simulink model "AN_Simulink_Model_v1_fil"  (R2019b)
settings: Solver=VariableStepAuto  StartTime=0.0  StopTime=testtime  RelTol=1e-3
InitFcn:
  | AN_InitFcn_Callback
StopFcn:
  | AN_StopFcn_Callback
undefined symbols (not defined in the file or in its folder): tdres
libraries: hdlmdlgenlib x193, simulink x4, fillib x1, dspsrcs4 x1
(part 1 of 6)
settings Model: Creator=mblun  LastModifiedBy=t96f346
settings OptimizationCC: BlockReduction=off  ConditionallyExecuteInputs=off  DefaultParameterBehavior=Inlined
settings DebuggingCC: AlgebraicLoopMsg=error  InheritedTsInSrcMsg=none  UnderSpecifiedDimensionMsg=warning
settings HardwareCC: ProdBitPerPointer=32  ProdBitPerSizeT=32  ProdBitPerPtrDiffT=32  ProdLargestAtomicFloat=None  ProdIntDivRoundTo=Undefined  ProdEndianess=Unspecified  ProdWordSize=32  ProdHWDeviceType=ASIC/FPGA->ASIC/FPGA  TargetBitPerPointer=64  TargetBitPerSizeT=64  TargetBitPerPtrDiffT=64  TargetLongLongMode=on  TargetIntDivRoundTo=Zero  TargetEndianess=LittleEndian  TargetWordSize=64  TargetHWDeviceType=Custom Processor->MATLAB Host Computer  ProdEqTarget=off
settings SFSimCC: CustomCodeUndefinedFunction=UseInterfaceOnly

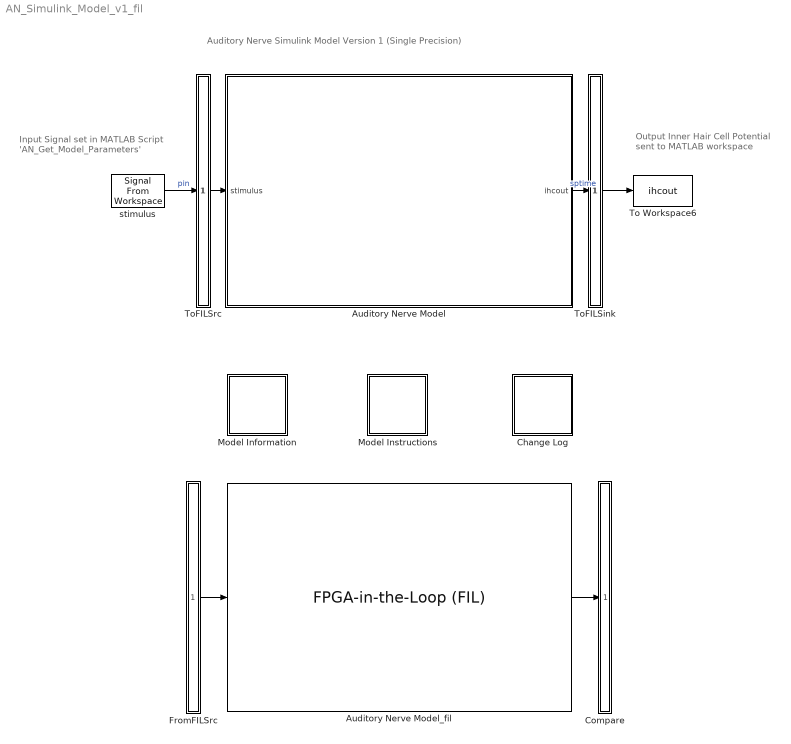
== system AN_Simulink_Model_v1_fil ==
  note: Input Signal set in MATLAB Script
      | 'AN_Get_Model_Parameters'
  note: Auditory Nerve Simulink Model Version 1 (Single Precision)
  note: Output Inner Hair Cell Potential
      | sent to MATLAB workspace
  Auditory Nerve Model : Subsystem
  Auditory Nerve Model_fil : fillib/FPGA-in-the-Loop (FIL)  ForceInterfaceUpdate=0.75839
      settings: SourceProductName=HDL Coder  SourceProductBaseCode=HD
  Change Log : Subsystem
  Compare : Subsystem
      mask Display: disp('')
  FromFILSrc : Subsystem
      mask Display: disp('')
  Model Information : Subsystem
  Model Instructions : Subsystem
  To Workspace6 : ToWorkspace  VariableName=ihcout  SampleTime=-1
      settings: Save2DSignal=2-D array (concatenate along first dimension)
  ToFILSink : Subsystem
      mask Display: disp('')
  ToFILSrc : Subsystem
      mask Display: disp('')
  "stimulus " : dspsrcs4/Signal From Workspace  X=RxSignal  Ts=tdres  nsamps=1  OutputAfterFinalValue=Setting to zero  ignoreOrWarnInputAndFrameLengths=off  OutputFrames=off
  wires:
  ToFILSrc/1(out1) -> Auditory Nerve Model/1(stimulus)
  Auditory Nerve Model/1(ihcout) -> ToFILSink/1(in1)  "sptime"
  "stimulus "/1 -> ToFILSrc/1(in1)  "pin"
  ToFILSink/1(out1) -> To Workspace6/1
  FromFILSrc/1(out1) -> Auditory Nerve Model_fil/1
  Auditory Nerve Model_fil/1 -> Compare/1(in1)

== system AN_Simulink_Model_v1_fil/Auditory Nerve Model ==
  stimulus : Inport  OutDataTypeStr=single  PortDimensions=1  SampleTime=2.08333333333333e-05
  C1 Chirp Filter : Subsystem
  C2 Wideband Filter : Subsystem
  CP Wideband Gammatone Filter : Subsystem
  Constant3 : Constant  Value=single(1.4316545724868774)  OutDataTypeStr=single  SampleTime=-1
  Constant4 : Constant  Value=single(0.0007758744177408516)  OutDataTypeStr=single  SampleTime=-1
  Middle Ear Filter : Subsystem
  Subsystem : Subsystem
  Subsystem1 : Subsystem
  ihcout : Outport  VectorParamsAs1DForOutWhenUnconnected=off
  wires:
  Subsystem1/1(tauc1) -> C1 Chirp Filter/2(tauc1)
  Subsystem/1(ihcout) -> ihcout/1
  Middle Ear Filter/1(output) -> C2 Wideband Filter/1(stimulus), C1 Chirp Filter/1(meout), CP Wideband Gammatone Filter/3(stimulus)
  Constant4/1 -> CP Wideband Gammatone Filter/2(tauwb)
  Constant3/1 -> CP Wideband Gammatone Filter/1(wbgain)
  CP Wideband Gammatone Filter/1(output1) -> Subsystem1/1(wbout)
  C2 Wideband Filter/1(output) -> Subsystem/1(C2filterout)
  C1 Chirp Filter/1(output) -> Subsystem/2(C1filterout)
  stimulus/1 -> Middle Ear Filter/1(stimulus)

== system AN_Simulink_Model_v1_fil/Change Log ==
  Change Log : simulink/Model-Wide Utilities/Model Info  Frame=on  DisplayStringWithTags=|  HorizontalTextAlignment=Left  LeftAlignmentValue=0.02
      | The following is the change log for the AN Simulink Model. Any major version changes should be 
      | documented and summarized below.
      | 
      | ------------------------------------------------------------------------------------------------------------------------------------
      | 
      | Version 1:
      | 	
      | 	- First Draft Version of Simulink Model by Matthew Blunt --- 08/07/2019
      | 
      | ------------------------------------------------------------------------------------------------------------------------------------
      | 
      | (Next Version Here)
      | 
      | 	- (Details and Changes Here)

== system AN_Simulink_Model_v1_fil/Compare ==
  in1 : Inport
  Assert_ihcout : Subsystem  mask{ToleranceValue=1e-07}
  CleanupScopes : Subsystem
      settings: OpenFcn=|
      | blkName = gcb; %self block
      | idx = regexp(blkName, '/CleanupScopes$', 'once');
      | blkParent = blkName(1:idx-1);
      | blks=find_system(blkParent, 'LookUnderMasks', 'all','blocktype', 'Scope');
      | for itr = 1:length(blks)
      | 	 hScopeCfg = get_param(blks{itr},'ScopeConfiguration');
      | 	 hScopeCfg.Visible = ~ hScopeCfg.Visible;
      | end
      | drawnow;
      mask Display: fprintf(message('hdlcoder:cosim:vnl_dblclick').getString());
  Enable : Subsystem
      settings: OpenFcn=|
      | blkName = gcb;
      | idx = regexp(blkName, '/Enable$', 'once');
      | blkParent = blkName(1:idx-1);
      | blks=find_system(blkParent, 'LookUnderMasks', 'all','blocktype', 'Assertion');
      | e = get_param(blks{1}, 'Enabled');
      | if strcmp(e, 'on'), f= 'off';, else, f = 'on';, end
      | for ii=1:length(blks), set_param(blks{ii}, 'Enabled', f);, end
      | set_param(gcb, 'MaskDisplay',['fprintf(message(''hdlcoder:cosim:vnl_dblclick_assertions'',','''',upper(e),'''',').getString())']);
      mask Display: fprintf(message('hdlcoder:cosim:vnl_dblclick_assertions','OFF').getString());
  wires:
  in1/1 -> Assert_ihcout/1(cosim)
  [out1] -> Assert_ihcout/2(dut)

== system AN_Simulink_Model_v1_fil/FromFILSrc ==
  dtc1 : DataTypeConversion  OutDataTypeStr=single  SaturateOnIntegerOverflow=on  RndMeth=Zero
  out1 : Outport
  wires:
  [in1] -> dtc1/1
  dtc1/1 -> out1/1

== system AN_Simulink_Model_v1_fil/Model Information ==
  "Model Information " : simulink/Model-Wide Utilities/Model Info  Frame=on  DisplayStringWithTags=|  HorizontalTextAlignment=Left  LeftAlignmentValue=0.02
      | Model Name: AN_Simulink_Model_v1
      | Created By: Matthew Blunt
      | Last Modification Date: 08/07/2019
      | Most Recently Modified By: Matthew Blunt
      | Model Version: 1
      | 
      | ------------------------------------------------------------------------------------------------------------------------------------
      | 
      | Description: This is a sample-based auditory nerve Simulink model, designed to closely replicate the 
      | auditory nerve model presented in the following publication:
      | 
      | 			Bruce, I.C., Erfani, Y., and Zilany, M.S.A. (2018). "A Phenomenological
      | 			model of the synapse between the inner hair cell and auditory nerve: 
      | 			Implications of limited neurotransmitter release sites," to appear in
      | 			Hearing Research. (Special Issue on "Computational Models in Hearing".)
      | 
      | It is important to also recognize the previous iterations of the phenomenological auditory 
      | nerve model, as they served as additional references during the design of the Simulink model.
      | 
      | ------------------------------------------------------------------------------------------------------------------------------------
      | 
      | This software was developed in conjunction with Flat Earth Inc
      | 
      | Copyright 2019 Flat Earth Inc
      | 
      | THE SOFTWARE IS PROVIDED "AS IS", WITHOUT WARRANTY OF ANY KIND, EXPRESS OR
      | IMPLIED, INCLUDING BUT NOT LIMITED TO THE WARRANTIES OF MERCHANTABILITY,
      | FITNESS FOR A PARTICULAR PURPOSE AND NONINFRINGEMENT. IN NO EVENT SHALL
      | THE AUTHORS OR COPYRIGHT HOLDERS BE LIABLE FOR ANY CLAIM, DAMAGES OR
      | OTHER LIABILITY, WHETHER IN AN ACTION OF CONTRACT, TORT OR OTHERWISE,
      | ARISING FROM, OUT OF OR IN CONNECTION WITH THE SOFTWARE OR THE USE OR
      | OTHER DEALINGS IN THE SOFTWARE.
      | 
      |    		Matthew Blunt
      |   		 Flat Earth Inc
      |    		985 Technology Blvd
      |    		Bozeman, MT 59718
      |    		support@flatearthinc.com

== system AN_Simulink_Model_v1_fil/Model Instructions ==
  "Model Instructions " : simulink/Model-Wide Utilities/Model Info  Frame=on  DisplayStringWithTags=|  HorizontalTextAlignment=Left  LeftAlignmentValue=0.02
      | The following is a full set of instructions outlining the necessary steps to be taken in order to run the 
      | AN Simulink Model. Instructions can also be found in the readme file found in the
      | AN_Simulink_Model_v1_Doubles folder.
      | 
      | ------------------------------------------------------------------------------------------------------------------------------------
      | 
      | ** Quick Start Instructions **
      | 
      | If the user desires to simply run the model as is, refer to the Quick Start
      | Instructions pdf, which gives a quick visual tutorial on running the Auditory
      | Nerve Simulink Model.
      | 
      | ------------------------------------------------------------------------------------------------------------------------------------
      | 
      | ** Modify Model Instructions **
      | 
      | If the user desires to make modifications to the model before runtime,
      | refer to the Modify Model Instructions pdf, which gives a quick visual
      | tutorial on modifying the Auditory Nerve Simulink Model.
      | 
      | ------------------------------------------------------------------------------------------------------------------------------------
      | 
      | ** Verify Model Instructions **
      | 
      | If the user desires to verify model functionality against the original 
      | model source code, instructions are listed below, as well as in the readme.txt file
      | 
      | 1. Make sure MATLAB R2019a and a compatible C compiler are downloaded on the
      | machine the model will be running on. The C compiler is needed for C functions
      | used in the test/verification process. The compiler used for testing was the
      | MinGW-w64 C/C++ Compiler. This can be easily accessed for free in the Add-On
      | Explorer found in the MATLAB home tab.
      | 
      | 2. Open the AN_Simulink_Model_v1_Doubles folder in MATLAB. This is necessary in
      | order for the Simulink model to interact with MATLAB.
      | 
      | 3. Edit model parameters, if necessary. This can be done by adjusting the
      | overall model parameters set in the AN_Set_Model_Parameters script, or adjusting
      | other parameters in the AN_Get_Model_Parameters script. Both scripts are found
      | in the AN_Simulink_Model_v1_Doubles folder.
      | 
      | 4. Set the 'verificationflag' boolean to 'true' in the AN_Set_Model_Parameters
      | script. This enables the model to run the comparison C/MATLAB source functions
      | which are compared to the Simulink Model.
      | 
      | 5. Run the model. This is done by simply clicking the green 'Run' button
      | located at the top panel of Simulink. In addition, the model can be stepped
      | through in increments, using the 'Step Through' button to the right of the
      | 'Run' button.

== system AN_Simulink_Model_v1_fil/ToFILSink ==
  in1 : Inport
  out1 : Outport
  tag scope: out1=global
  wires:
  in1/1 -> out1/1, [out1]

== system AN_Simulink_Model_v1_fil/ToFILSrc ==
  in1 : Inport
  out1 : Outport
  tag scope: in1=global
  wires:
  in1/1 -> out1/1, [in1]

== system AN_Simulink_Model_v1_fil/Auditory Nerve Model/C1 Chirp Filter ==
  meout : Inport  OutDataTypeStr=single  PortDimensions=1  SampleTime=2.08333333333333e-05
  tauc1 : Inport  Port=2  OutDataTypeStr=single  PortDimensions=1  SampleTime=2.08333333333333e-05
  C1 FIlter : Subsystem
  Calculate C1filterout : Subsystem
  Calculate rsigma : Subsystem
  Get C1 Coefficients : Subsystem
  To Workspace2 : ToWorkspace  VariableName=rsigma  SampleTime=-1
      settings: Save2DSignal=2-D array (concatenate along first dimension)
  output : Outport  VectorParamsAs1DForOutWhenUnconnected=off
  wires:
  Get C1 Coefficients/15(a1(5)) -> C1 FIlter/16(a1(5))
  Get C1 Coefficients/14(a1(3)) -> C1 FIlter/15(a1(3))
  Get C1 Coefficients/13(a1(1)) -> C1 FIlter/14(a1(1))
  Get C1 Coefficients/12(a2(1)) -> C1 FIlter/13(a2(1))
  Get C1 Coefficients/11(a2(3)) -> C1 FIlter/12(a2(3))
  Get C1 Coefficients/10(a2(5)) -> C1 FIlter/11(a2(5))
  Get C1 Coefficients/9(b2(1)) -> C1 FIlter/10(b2(1))
  Get C1 Coefficients/8(b2(3)) -> C1 FIlter/9(b2(3))
  Get C1 Coefficients/7(b2(5)) -> C1 FIlter/8(b2(5))
  Get C1 Coefficients/6(b1(1)) -> C1 FIlter/7(b1(1))
  Get C1 Coefficients/5(b1(3)) -> C1 FIlter/6(b1(3))
  Get C1 Coefficients/4(b1(5)) -> C1 FIlter/5(b1(5))
  Get C1 Coefficients/3(b0(1)) -> C1 FIlter/4(b0(1))
  Get C1 Coefficients/2(b0(3)) -> C1 FIlter/3(b0(3))
  Get C1 Coefficients/1(b0(5)) -> C1 FIlter/2(b0(5))
  Calculate rsigma/1(rsigma) -> Get C1 Coefficients/1(rsigma), To Workspace2/1
  Calculate C1filterout/1(C1filterout) -> output/1
  C1 FIlter/1(Out1) -> Calculate C1filterout/1(C1filterouttmp)
  tauc1/1 -> Calculate rsigma/1(tauc1)
  meout/1 -> C1 FIlter/1(meout)

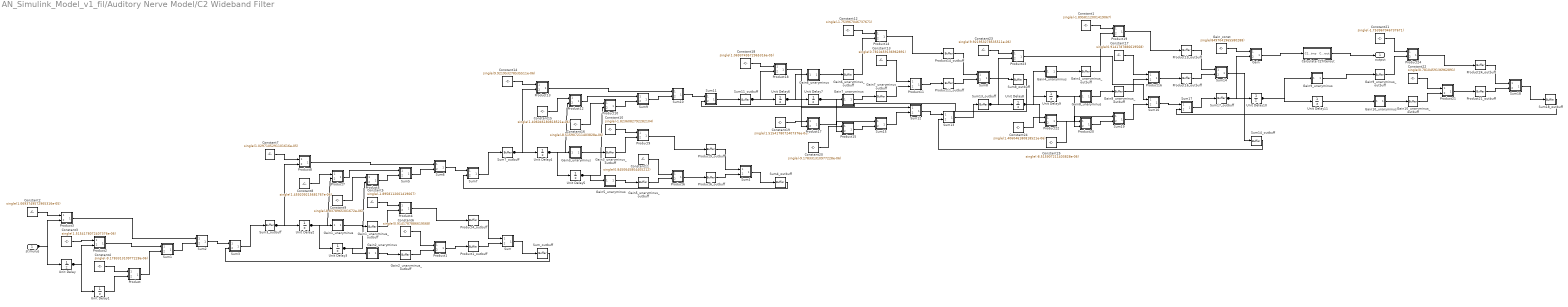
== system AN_Simulink_Model_v1_fil/Auditory Nerve Model/C2 Wideband Filter ==
  stimulus : Inport  OutDataTypeStr=single  PortDimensions=1  SampleTime=2.08333333333333e-05
  Calculate C2filterout : Subsystem
  Constant1 : Constant  Value=single(-1.8958112001419067)  OutDataTypeStr=single  SampleTime=-1
  Constant10 : Constant  Value=single(-1.8236082792282104)  OutDataTypeStr=single  SampleTime=-1
  Constant11 : Constant  Value=single(0.8450645804405212)  OutDataTypeStr=single  SampleTime=-1
  Constant12 : Constant  Value=single(-1.753967046737671)  OutDataTypeStr=single  SampleTime=-1
  Constant13 : Constant  Value=single(0.7810459136962891)  OutDataTypeStr=single  SampleTime=-1
  Constant14 : Constant  Value=single(9.921953278535511e-06)  OutDataTypeStr=single  SampleTime=-1
  Constant15 : Constant  Value=single(1.406046180818521e-06)  OutDataTypeStr=single  SampleTime=-1
  Constant16 : Constant  Value=single(-8.515907211403828e-06)  OutDataTypeStr=single  SampleTime=-1
  Constant17 : Constant  Value=single(0.9141787886619568)  OutDataTypeStr=single  SampleTime=-1
  Constant18 : Constant  Value=single(1.0693749572965316e-05)  OutDataTypeStr=single  SampleTime=-1
  Constant19 : Constant  Value=single(1.5154178072407376e-06)  OutDataTypeStr=single  SampleTime=-1
  Constant2 : Constant  Value=single(1.0693749572965316e-05)  OutDataTypeStr=single  SampleTime=-1
  Constant20 : Constant  Value=single(-9.178331310977228e-06)  OutDataTypeStr=single  SampleTime=-1
  Constant21 : Constant  Value=single(-1.753967046737671)  OutDataTypeStr=single  SampleTime=-1
  Constant22 : Constant  Value=single(0.7810459136962891)  OutDataTypeStr=single  SampleTime=-1
  Constant23 : Constant  Value=single(9.921953278535511e-06)  OutDataTypeStr=single  SampleTime=-1
  Constant24 : Constant  Value=single(1.406046180818521e-06)  OutDataTypeStr=single  SampleTime=-1
  Constant25 : Constant  Value=single(-8.515907211403828e-06)  OutDataTypeStr=single  SampleTime=-1
  Constant3 : Constant  Value=single(1.5154178072407376e-06)  OutDataTypeStr=single  SampleTime=-1
  Constant4 : Constant  Value=single(-9.178331310977228e-06)  OutDataTypeStr=single  SampleTime=-1
  Constant5 : Constant  Value=single(-1.8958112001419067)  OutDataTypeStr=single  SampleTime=-1
  Constant6 : Constant  Value=single(0.9141787886619568)  OutDataTypeStr=single  SampleTime=-1
  Constant7 : Constant  Value=single(1.0297105291101616e-05)  OutDataTypeStr=single  SampleTime=-1
  Constant8 : Constant  Value=single(1.459209215681767e-06)  OutDataTypeStr=single  SampleTime=-1
  Constant9 : Constant  Value=single(-8.8378965301672e-06)  OutDataTypeStr=single  SampleTime=-1
  Gain : Subsystem
      mask Display: disp('NFP\nmul');
  Gain10_unaryminus : Subsystem
      mask Display: disp('NFP\numinus');
  Gain10_unaryminus_outbuff : hdlmdlgenlib/Buffer
      settings: SourceProductName=Simulink  SourceProductBaseCode=SL
  Gain1_unaryminus : Subsystem
      mask Display: disp('NFP\numinus');
  Gain1_unaryminus_outbuff : hdlmdlgenlib/Buffer
      settings: SourceProductName=Simulink  SourceProductBaseCode=SL
  Gain2_unaryminus : Subsystem
      mask Display: disp('NFP\numinus');
  Gain2_unaryminus_outbuff : hdlmdlgenlib/Buffer
      settings: SourceProductName=Simulink  SourceProductBaseCode=SL
  Gain3_unaryminus : Subsystem
      mask Display: disp('NFP\numinus');
  Gain3_unaryminus_outbuff : hdlmdlgenlib/Buffer
      settings: SourceProductName=Simulink  SourceProductBaseCode=SL
  Gain4_unaryminus : Subsystem
      mask Display: disp('NFP\numinus');
  Gain4_unaryminus_outbuff : hdlmdlgenlib/Buffer
      settings: SourceProductName=Simulink  SourceProductBaseCode=SL
  Gain5_unaryminus : Subsystem
      mask Display: disp('NFP\numinus');
  Gain5_unaryminus_outbuff : hdlmdlgenlib/Buffer
      settings: SourceProductName=Simulink  SourceProductBaseCode=SL
  Gain6_unaryminus : Subsystem
      mask Display: disp('NFP\numinus');
  Gain6_unaryminus_outbuff : hdlmdlgenlib/Buffer
      settings: SourceProductName=Simulink  SourceProductBaseCode=SL
  Gain7_unaryminus : Subsystem
      mask Display: disp('NFP\numinus');
  Gain7_unaryminus_outbuff : hdlmdlgenlib/Buffer
      settings: SourceProductName=Simulink  SourceProductBaseCode=SL
  Gain8_unaryminus : Subsystem
      mask Display: disp('NFP\numinus');
  Gain8_unaryminus_outbuff : hdlmdlgenlib/Buffer
      settings: SourceProductName=Simulink  SourceProductBaseCode=SL
  Gain9_unaryminus : Subsystem
      mask Display: disp('NFP\numinus');
  Gain9_unaryminus_outbuff : hdlmdlgenlib/Buffer
      settings: SourceProductName=Simulink  SourceProductBaseCode=SL
  Gain_const : Constant  Value=single(8497041965580288)  OutDataTypeStr=single  SampleTime=-1
  Product : Subsystem
      mask Display: disp('NFP\nmul');
  Product1 : Subsystem
      mask Display: disp('NFP\nmul');
  Product10 : Subsystem
      mask Display: disp('NFP\nmul');
  Product11 : Subsystem
      mask Display: disp('NFP\nmul');
  Product11_outbuff : hdlmdlgenlib/Buffer
      settings: SourceProductName=Simulink  SourceProductBaseCode=SL
  Product12 : Subsystem
      mask Display: disp('NFP\nmul');
  Product13 : Subsystem
      mask Display: disp('NFP\nmul');
  Product14 : Subsystem
      mask Display: disp('NFP\nmul');
  Product14_outbuff : hdlmdlgenlib/Buffer
      settings: SourceProductName=Simulink  SourceProductBaseCode=SL
  Product15 : Subsystem
      mask Display: disp('NFP\nmul');
  Product16 : Subsystem
      mask Display: disp('NFP\nmul');
  Product16_outbuff : hdlmdlgenlib/Buffer
      settings: SourceProductName=Simulink  SourceProductBaseCode=SL
  Product17 : Subsystem
      mask Display: disp('NFP\nmul');
  Product18 : Subsystem
      mask Display: disp('NFP\nmul');
  Product19 : Subsystem
      mask Display: disp('NFP\nmul');
  Product19_outbuff : hdlmdlgenlib/Buffer
      settings: SourceProductName=Simulink  SourceProductBaseCode=SL
  Product1_outbuff : hdlmdlgenlib/Buffer
      settings: SourceProductName=Simulink  SourceProductBaseCode=SL
  Product2 : Subsystem
      mask Display: disp('NFP\nmul');
  Product20 : Subsystem
      mask Display: disp('NFP\nmul');
  Product21 : Subsystem
      mask Display: disp('NFP\nmul');
  Product21_outbuff : hdlmdlgenlib/Buffer
      settings: SourceProductName=Simulink  SourceProductBaseCode=SL
  Product22 : Subsystem
      mask Display: disp('NFP\nmul');
  Product23 : Subsystem
      mask Display: disp('NFP\nmul');
  Product24 : Subsystem
      mask Display: disp('NFP\nmul');
  Product24_outbuff : hdlmdlgenlib/Buffer
      settings: SourceProductName=Simulink  SourceProductBaseCode=SL
  Product3 : Subsystem
      mask Display: disp('NFP\nmul');
  Product4 : Subsystem
      mask Display: disp('NFP\nmul');
  Product4_outbuff : hdlmdlgenlib/Buffer
      settings: SourceProductName=Simulink  SourceProductBaseCode=SL
  Product5 : Subsystem
      mask Display: disp('NFP\nmul');
  Product6 : Subsystem
      mask Display: disp('NFP\nmul');
  Product6_outbuff : hdlmdlgenlib/Buffer
      settings: SourceProductName=Simulink  SourceProductBaseCode=SL
  Product7 : Subsystem
      mask Display: disp('NFP\nmul');
  Product8 : Subsystem
      mask Display: disp('NFP\nmul');
  Product9 : Subsystem
      mask Display: disp('NFP\nmul');
  Product9_outbuff : hdlmdlgenlib/Buffer
      settings: SourceProductName=Simulink  SourceProductBaseCode=SL
  Sum : Subsystem
      mask Display: disp('NFP\nadd');
  Sum1 : Subsystem
      mask Display: disp('NFP\nadd');
  Sum10 : Subsystem
      mask Display: disp('NFP\nadd');
  Sum11 : Subsystem
      mask Display: disp('NFP\nadd');
  Sum11_outbuff : hdlmdlgenlib/Buffer
      settings: SourceProductName=Simulink  SourceProductBaseCode=SL
  Sum12 : Subsystem
      mask Display: disp('NFP\nadd');
  Sum13 : Subsystem
      mask Display: disp('NFP\nadd');
  Sum13_outbuff : hdlmdlgenlib/Buffer
      settings: SourceProductName=Simulink  SourceProductBaseCode=SL
  Sum14 : Subsystem
      mask Display: disp('NFP\nadd');
  Sum14_outbuff : hdlmdlgenlib/Buffer
      settings: SourceProductName=Simulink  SourceProductBaseCode=SL
  Sum15 : Subsystem
      mask Display: disp('NFP\nadd');
  Sum16 : Subsystem
      mask Display: disp('NFP\nadd');
  Sum17 : Subsystem
      mask Display: disp('NFP\nadd');
  Sum17_outbuff : hdlmdlgenlib/Buffer
      settings: SourceProductName=Simulink  SourceProductBaseCode=SL
  Sum18 : Subsystem
      mask Display: disp('NFP\nadd');
  Sum18_outbuff : hdlmdlgenlib/Buffer
      settings: SourceProductName=Simulink  SourceProductBaseCode=SL
  Sum19 : Subsystem
      mask Display: disp('NFP\nadd');
  Sum2 : Subsystem
      mask Display: disp('NFP\nadd');
  Sum3 : Subsystem
      mask Display: disp('NFP\nadd');
  Sum3_outbuff : hdlmdlgenlib/Buffer
      settings: SourceProductName=Simulink  SourceProductBaseCode=SL
  Sum4 : Subsystem
      mask Display: disp('NFP\nadd');
  Sum4_outbuff : hdlmdlgenlib/Buffer
      settings: SourceProductName=Simulink  SourceProductBaseCode=SL
  Sum5 : Subsystem
      mask Display: disp('NFP\nadd');
  Sum6 : Subsystem
      mask Display: disp('NFP\nadd');
  Sum7 : Subsystem
      mask Display: disp('NFP\nadd');
  Sum7_outbuff : hdlmdlgenlib/Buffer
      settings: SourceProductName=Simulink  SourceProductBaseCode=SL
  Sum8 : Subsystem
      mask Display: disp('NFP\nadd');
  Sum8_outbuff : hdlmdlgenlib/Buffer
      settings: SourceProductName=Simulink  SourceProductBaseCode=SL
  Sum9 : Subsystem
      mask Display: disp('NFP\nadd');
  Sum_outbuff : hdlmdlgenlib/Buffer
      settings: SourceProductName=Simulink  SourceProductBaseCode=SL
  Unit Delay{,1..11} (12 alike) : UnitDelay  InitialCondition=single(0)  SampleTime=2.08333333333333e-05
  output : Outport  VectorParamsAs1DForOutWhenUnconnected=off
  wires:
  Gain/1(Out1) -> Calculate C2filterout/1(C2filterouttmp)
  Sum9/1(Out1) -> Sum10/2(In2)
  Sum8/1(Out1) -> Sum8_outbuff/1
  Sum7/1(Out1) -> Sum7_outbuff/1
  Sum6/1(Out1) -> Sum7/1(In1)
  Sum5/1(Out1) -> Sum6/2(In2)
  Sum4/1(Out1) -> Sum4_outbuff/1
  Sum3/1(Out1) -> Sum3_outbuff/1
  Sum2/1(Out1) -> Sum3/1(In1)
  Sum19/1(Out1) -> Sum16/2(In2)
  Sum18/1(Out1) -> Sum18_outbuff/1
  Sum17/1(Out1) -> Sum17_outbuff/1
  Sum16/1(Out1) -> Sum17/1(In1)
  Sum15/1(Out1) -> Sum12/2(In2)
  Sum14/1(Out1) -> Sum14_outbuff/1
  Sum13/1(Out1) -> Sum13_outbuff/1
  Sum12/1(Out1) -> Sum13/1(In1)
  Sum11/1(Out1) -> Sum11_outbuff/1
  Sum10/1(Out1) -> Sum11/1(In1)
  Sum1/1(Out1) -> Sum2/2(In2)
  Sum/1(Out1) -> Sum_outbuff/1
  Product9/1(Out1) -> Product9_outbuff/1
  Product8/1(Out1) -> Sum6/1(In1)
  Product7/1(Out1) -> Sum5/1(In1)
  Product6/1(Out1) -> Product6_outbuff/1
  Product5/1(Out1) -> Sum5/2(In2)
  Product4/1(Out1) -> Product4_outbuff/1
  Product3/1(Out1) -> Sum2/1(In1)
  Product24/1(Out1) -> Product24_outbuff/1
  Product23/1(Out1) -> Sum16/1(In1)
  Product22/1(Out1) -> Sum19/1(In1)
  Product21/1(Out1) -> Product21_outbuff/1
  Product20/1(Out1) -> Sum19/2(In2)
  Product2/1(Out1) -> Sum1/1(In1)
  Product19/1(Out1) -> Product19_outbuff/1
  Product18/1(Out1) -> Sum12/1(In1)
  Product17/1(Out1) -> Sum15/1(In1)
  Product16/1(Out1) -> Product16_outbuff/1
  Product15/1(Out1) -> Sum15/2(In2)
  Product14/1(Out1) -> Product14_outbuff/1
  Product13/1(Out1) -> Sum10/1(In1)
  Product12/1(Out1) -> Sum9/1(In1)
  Product11/1(Out1) -> Product11_outbuff/1
  Product10/1(Out1) -> Sum9/2(In2)
  Product1/1(Out1) -> Product1_outbuff/1
  Product/1(Out1) -> Sum1/2(In2)
  Gain9_unaryminus/1(Out1) -> Gain9_unaryminus_outbuff/1
  Gain8_unaryminus/1(Out1) -> Gain8_unaryminus_outbuff/1
  Gain7_unaryminus/1(Out1) -> Gain7_unaryminus_outbuff/1
  Gain6_unaryminus/1(Out1) -> Gain6_unaryminus_outbuff/1
  Gain5_unaryminus/1(Out1) -> Gain5_unaryminus_outbuff/1
  Gain4_unaryminus/1(Out1) -> Gain4_unaryminus_outbuff/1
  Gain3_unaryminus/1(Out1) -> Gain3_unaryminus_outbuff/1
  Gain2_unaryminus/1(Out1) -> Gain2_unaryminus_outbuff/1
  Gain10_unaryminus/1(Out1) -> Gain10_unaryminus_outbuff/1
  Gain1_unaryminus/1(Out1) -> Gain1_unaryminus_outbuff/1
  Gain_const/1 -> Gain/1(In1)
  Unit Delay9/1 -> Gain8_unaryminus/1(In1), Product20/2(In2)
  Unit Delay8/1 -> Unit Delay9/1, Gain4_unaryminus/1(In1), Product22/2(In2)
  Unit Delay7/1 -> Gain7_unaryminus/1(In1), Product15/2(In2)
  Unit Delay6/1 -> Unit Delay7/1, Gain6_unaryminus/1(In1), Product17/2(In2)
  Unit Delay5/1 -> Gain5_unaryminus/1(In1), Product10/2(In2)
  Unit Delay4/1 -> Unit Delay5/1, Gain3_unaryminus/1(In1), Product12/2(In2)
  Unit Delay3/1 -> Gain2_unaryminus/1(In1), Product5/2(In2)
  Unit Delay2/1 -> Unit Delay3/1, Gain1_unaryminus/1(In1), Product7/2(In2)
  Unit Delay11/1 -> Gain10_unaryminus/1(In1)
  Unit Delay10/1 -> Unit Delay11/1, Gain9_unaryminus/1(In1)
  Unit Delay1/1 -> Product/2(In2)
  Unit Delay/1 -> Unit Delay1/1, Product2/2(In2)
  Sum8_outbuff/1 -> Sum11/2(In2)
  Sum7_outbuff/1 -> Unit Delay4/1, Product13/2(In2)
  Sum4_outbuff/1 -> Sum7/2(In2)
  Sum3_outbuff/1 -> Unit Delay2/1, Product8/2(In2)
  Sum18_outbuff/1 -> Sum17/2(In2)
  Sum17_outbuff/1 -> Unit Delay10/1, Gain/2(In2)
  Sum14_outbuff/1 -> Sum13/2(In2)
  Sum13_outbuff/1 -> Unit Delay8/1, Product23/2(In2)
  Sum11_outbuff/1 -> Unit Delay6/1, Product18/2(In2)
  Sum_outbuff/1 -> Sum3/2(In2)
  Product9_outbuff/1 -> Sum4/1(In1)
  Product6_outbuff/1 -> Sum4/2(In2)
  Product4_outbuff/1 -> Sum/1(In1)
  Product24_outbuff/1 -> Sum18/1(In1)
  Product21_outbuff/1 -> Sum18/2(In2)
  Product19_outbuff/1 -> Sum14/1(In1)
  Product16_outbuff/1 -> Sum14/2(In2)
  Product14_outbuff/1 -> Sum8/1(In1)
  Product11_outbuff/1 -> Sum8/2(In2)
  Product1_outbuff/1 -> Sum/2(In2)
  Gain9_unaryminus_outbuff/1 -> Product24/2(In2)
  Gain8_unaryminus_outbuff/1 -> Product16/2(In2)
  Gain7_unaryminus_outbuff/1 -> Product11/2(In2)
  Gain6_unaryminus_outbuff/1 -> Product14/2(In2)
  Gain5_unaryminus_outbuff/1 -> Product6/2(In2)
  Gain4_unaryminus_outbuff/1 -> Product19/2(In2)
  Gain3_unaryminus_outbuff/1 -> Product9/2(In2)
  Gain2_unaryminus_outbuff/1 -> Product1/2(In2)
  Gain10_unaryminus_outbuff/1 -> Product21/2(In2)
  Gain1_unaryminus_outbuff/1 -> Product4/2(In2)
  Constant9/1 -> Product5/1(In1)
  Constant8/1 -> Product7/1(In1)
  Constant7/1 -> Product8/1(In1)
  Constant6/1 -> Product1/1(In1)
  Constant5/1 -> Product4/1(In1)
  Constant4/1 -> Product/1(In1)
  Constant3/1 -> Product2/1(In1)
  Constant25/1 -> Product20/1(In1)
  Constant24/1 -> Product22/1(In1)
  Constant23/1 -> Product23/1(In1)
  Constant22/1 -> Product21/1(In1)
  Constant21/1 -> Product24/1(In1)
  Constant20/1 -> Product15/1(In1)
  Constant2/1 -> Product3/1(In1)
  Constant19/1 -> Product17/1(In1)
  Constant18/1 -> Product18/1(In1)
  Constant17/1 -> Product16/1(In1)
  Constant16/1 -> Product10/1(In1)
  Constant15/1 -> Product12/1(In1)
  Constant14/1 -> Product13/1(In1)
  Constant13/1 -> Product11/1(In1)
  Constant12/1 -> Product14/1(In1)
  Constant11/1 -> Product6/1(In1)
  Constant10/1 -> Product9/1(In1)
  Constant1/1 -> Product19/1(In1)
  Calculate C2filterout/1(C2filterout) -> output/1
  stimulus/1 -> Unit Delay/1, Product3/2(In2)

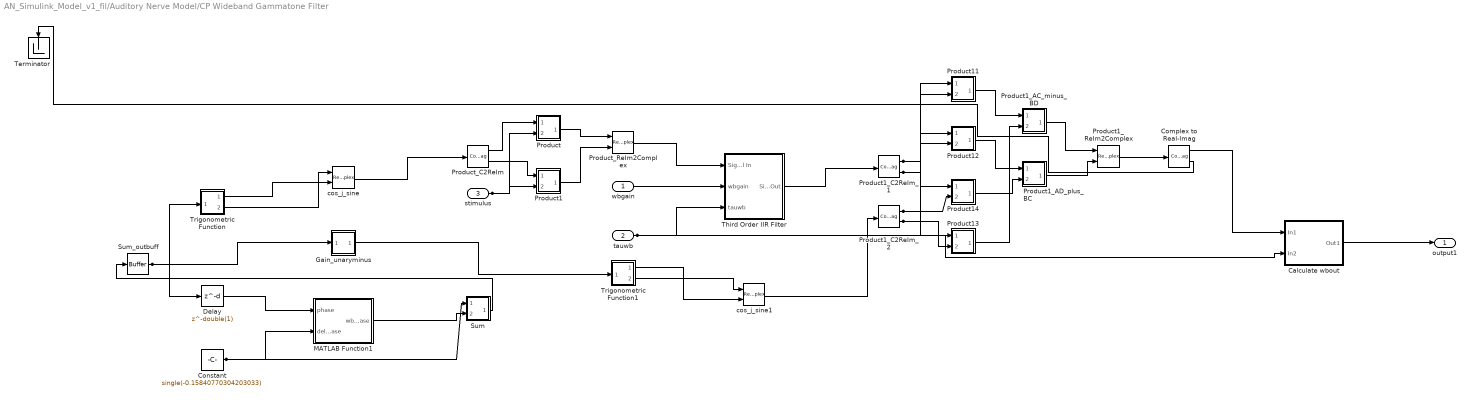
== system AN_Simulink_Model_v1_fil/Auditory Nerve Model/CP Wideband Gammatone Filter ==
  wbgain : Inport  OutDataTypeStr=single  PortDimensions=1  SampleTime=2.08333333333333e-05
  tauwb : Inport  Port=2  OutDataTypeStr=single  PortDimensions=1  SampleTime=2.08333333333333e-05
  stimulus : Inport  Port=3  OutDataTypeStr=single  PortDimensions=1  SampleTime=2.08333333333333e-05
  Calculate wbout : Subsystem
  Complex to Real-Imag : ComplexToRealImag  SampleTime=2.08333333333333e-05
  Constant : Constant  Value=single(-0.15840770304203033)  OutDataTypeStr=single  SampleTime=-1
  Delay : Delay  DelayLength=double(1)  InitialCondition=0  SampleTime=2.08333333333333e-05
  Gain_unaryminus : Subsystem
      mask Display: disp('NFP\numinus');
  MATLAB Function1 : Subsystem
  Product : Subsystem
      mask Display: disp('NFP\nmul');
  Product1 : Subsystem
      mask Display: disp('NFP\nmul');
  Product11 : Subsystem
      mask Display: disp('NFP\nmul');
  Product12 : Subsystem
      mask Display: disp('NFP\nmul');
  Product13 : Subsystem
      mask Display: disp('NFP\nmul');
  Product14 : Subsystem
      mask Display: disp('NFP\nmul');
  Product1_AC_minus_BD : Subsystem
      mask Display: disp('NFP\nadd');
  Product1_AD_plus_BC : Subsystem
      mask Display: disp('NFP\nadd');
  Product1_C2ReIm_1 : ComplexToRealImag  SampleTime=2.08333333333333e-05
  Product1_C2ReIm_2 : ComplexToRealImag  SampleTime=2.08333333333333e-05
  Product1_ReIm2Complex : RealImagToComplex  SampleTime=2.08333333333333e-05
  Product_C2ReIm : ComplexToRealImag  SampleTime=2.08333333333333e-05
  Product_ReIm2Complex : RealImagToComplex  SampleTime=2.08333333333333e-05
  Sum : Subsystem
      mask Display: disp('NFP\nadd');
  Sum_outbuff : hdlmdlgenlib/Buffer
      settings: SourceProductName=Simulink  SourceProductBaseCode=SL
  Terminator : Terminator
  Third Order IIR Filter : Subsystem
  Trigonometric Function : Subsystem
      mask Display: disp('NFP\ntrig2');
  Trigonometric Function1 : Subsystem
      mask Display: disp('NFP\ntrig2');
  cos_j_sine : RealImagToComplex  ConstantPart=single(0)  SampleTime=2.08333333333333e-05
  cos_j_sine1 : RealImagToComplex  ConstantPart=single(0)  SampleTime=2.08333333333333e-05
  output1 : Outport  VectorParamsAs1DForOutWhenUnconnected=off
  wires:
  Product1_AD_plus_BC/1(Out1) -> Product1_ReIm2Complex/2
  Product1_AC_minus_BD/1(Out1) -> Product1_ReIm2Complex/1
  Product14/1(Out1) -> Product1_AD_plus_BC/2(In2)
  Product13/1(Out1) -> Product1_AC_minus_BD/2(In2)
  Product12/1(Out1) -> Product1_AD_plus_BC/1(In1)
  Product11/1(Out1) -> Product1_AC_minus_BD/1(In1)
  Product1/1(Out1) -> Product_ReIm2Complex/2
  Product/1(Out1) -> Product_ReIm2Complex/1
  Trigonometric Function1/2(Out2) -> cos_j_sine1/1
  Trigonometric Function1/1(Out1) -> cos_j_sine1/2
  Trigonometric Function/2(Out2) -> cos_j_sine/1
  Trigonometric Function/1(Out1) -> cos_j_sine/2
  Sum/1(Out1) -> Sum_outbuff/1
  Gain_unaryminus/1(Out1) -> Trigonometric Function1/1(In1)
  Product1_C2ReIm_2/2 -> Product12/2(In2), Product13/2(In2)
  Product1_C2ReIm_2/1 -> Product11/2(In2), Product14/2(In2)
  Product1_C2ReIm_1/2 -> Product13/1(In1), Product14/1(In1)
  Product1_C2ReIm_1/1 -> Product11/1(In1), Product12/1(In1)
  Product_C2ReIm/2 -> Product1/1(In1)
  Product_C2ReIm/1 -> Product/1(In1)
  cos_j_sine1/1 -> Product1_C2ReIm_2/1
  cos_j_sine/1 -> Product_C2ReIm/1
  Third Order IIR Filter/1(Signal Out) -> Product1_C2ReIm_1/1
  Sum_outbuff/1 -> Delay/1, Gain_unaryminus/1(In1), Trigonometric Function/1(In1)
  Product1_ReIm2Complex/1 -> Complex to Real-Imag/1
  Product_ReIm2Complex/1 -> Third Order IIR Filter/1(Signal In)
  MATLAB Function1/1(wbphase) -> Sum/2(In2)
  Delay/1 -> MATLAB Function1/1(phase)
  Constant/1 -> MATLAB Function1/2(delta_phase), Sum/1(In1)
  Complex to Real-Imag/2 -> Terminator/1
  Complex to Real-Imag/1 -> Calculate wbout/1(In1)
  Calculate wbout/1(Out1) -> output1/1
  stimulus/1 -> Product/2(In2), Product1/2(In2)
  tauwb/1 -> Third Order IIR Filter/3(tauwb), Calculate wbout/2(In2)
  wbgain/1 -> Third Order IIR Filter/2(wbgain)

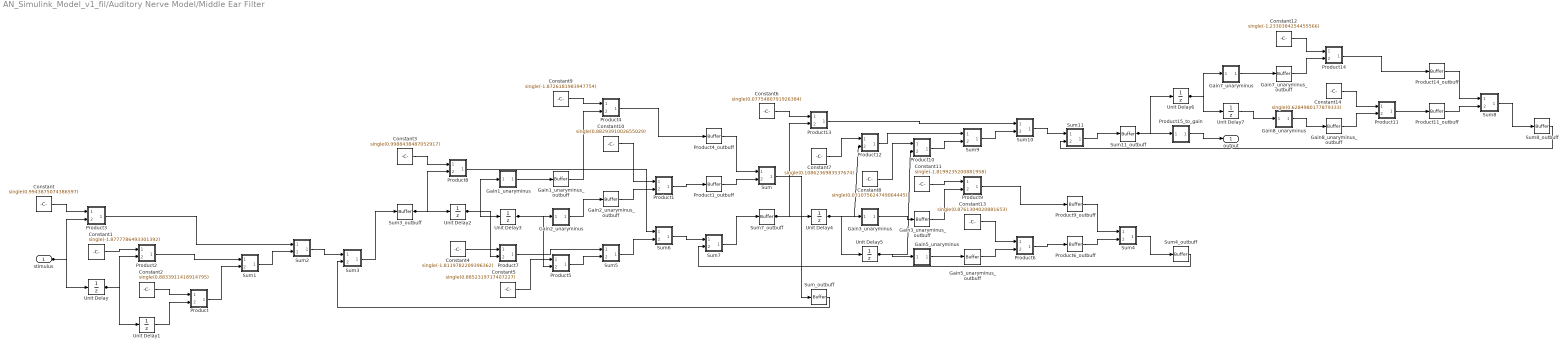
== system AN_Simulink_Model_v1_fil/Auditory Nerve Model/Middle Ear Filter ==
  stimulus : Inport  OutDataTypeStr=single  PortDimensions=1  SampleTime=2.08333333333333e-05
  Constant : Constant  Value=single(0.9943875074386597)  OutDataTypeStr=single  SampleTime=-1
  Constant1 : Constant  Value=single(-1.8777786493301392)  OutDataTypeStr=single  SampleTime=-1
  Constant10 : Constant  Value=single(0.8829391002655029)  OutDataTypeStr=single  SampleTime=-1
  Constant11 : Constant  Value=single(-1.8199235200881958)  OutDataTypeStr=single  SampleTime=-1
  Constant12 : Constant  Value=single(-1.2330384254455566)  OutDataTypeStr=single  SampleTime=-1
  Constant13 : Constant  Value=single(0.8761304020881653)  OutDataTypeStr=single  SampleTime=-1
  Constant14 : Constant  Value=single(0.6284980177879333)  OutDataTypeStr=single  SampleTime=-1
  Constant2 : Constant  Value=single(0.8833911418914795)  OutDataTypeStr=single  SampleTime=-1
  Constant3 : Constant  Value=single(0.9988438487052917)  OutDataTypeStr=single  SampleTime=-1
  Constant4 : Constant  Value=single(-1.8119782209396362)  OutDataTypeStr=single  SampleTime=-1
  Constant5 : Constant  Value=single(0.8852319717407227)  OutDataTypeStr=single  SampleTime=-1
  Constant6 : Constant  Value=single(0.0775480791926384)  OutDataTypeStr=single  SampleTime=-1
  Constant7 : Constant  Value=single(0.1086236983537674)  OutDataTypeStr=single  SampleTime=-1
  Constant8 : Constant  Value=single(0.031075624749064445)  OutDataTypeStr=single  SampleTime=-1
  Constant9 : Constant  Value=single(-1.8726181983947754)  OutDataTypeStr=single  SampleTime=-1
  Gain1_unaryminus : Subsystem
      mask Display: disp('NFP\numinus');
  Gain1_unaryminus_outbuff : hdlmdlgenlib/Buffer
      settings: SourceProductName=Simulink  SourceProductBaseCode=SL
  Gain2_unaryminus : Subsystem
      mask Display: disp('NFP\numinus');
  Gain2_unaryminus_outbuff : hdlmdlgenlib/Buffer
      settings: SourceProductName=Simulink  SourceProductBaseCode=SL
  Gain3_unaryminus : Subsystem
      mask Display: disp('NFP\numinus');
  Gain3_unaryminus_outbuff : hdlmdlgenlib/Buffer
      settings: SourceProductName=Simulink  SourceProductBaseCode=SL
  Gain5_unaryminus : Subsystem
      mask Display: disp('NFP\numinus');
  Gain5_unaryminus_outbuff : hdlmdlgenlib/Buffer
      settings: SourceProductName=Simulink  SourceProductBaseCode=SL
  Gain7_unaryminus : Subsystem
      mask Display: disp('NFP\numinus');
  Gain7_unaryminus_outbuff : hdlmdlgenlib/Buffer
      settings: SourceProductName=Simulink  SourceProductBaseCode=SL
  Gain8_unaryminus : Subsystem
      mask Display: disp('NFP\numinus');
  Gain8_unaryminus_outbuff : hdlmdlgenlib/Buffer
      settings: SourceProductName=Simulink  SourceProductBaseCode=SL
  Product : Subsystem
      mask Display: disp('NFP\nmul');
  Product1 : Subsystem
      mask Display: disp('NFP\nmul');
  Product10 : Subsystem
      mask Display: disp('NFP\nmul');
  Product11 : Subsystem
      mask Display: disp('NFP\nmul');
  Product11_outbuff : hdlmdlgenlib/Buffer
      settings: SourceProductName=Simulink  SourceProductBaseCode=SL
  Product12 : Subsystem
      mask Display: disp('NFP\nmul');
  Product13 : Subsystem
      mask Display: disp('NFP\nmul');
  Product14 : Subsystem
      mask Display: disp('NFP\nmul');
  Product14_outbuff : hdlmdlgenlib/Buffer
      settings: SourceProductName=Simulink  SourceProductBaseCode=SL
  Product15_to_gain : Subsystem
      mask Display: disp('NFP\ngain_pow2');
  Product1_outbuff : hdlmdlgenlib/Buffer
      settings: SourceProductName=Simulink  SourceProductBaseCode=SL
  Product2 : Subsystem
      mask Display: disp('NFP\nmul');
  Product3 : Subsystem
      mask Display: disp('NFP\nmul');
  Product4 : Subsystem
      mask Display: disp('NFP\nmul');
  Product4_outbuff : hdlmdlgenlib/Buffer
      settings: SourceProductName=Simulink  SourceProductBaseCode=SL
  Product5 : Subsystem
      mask Display: disp('NFP\nmul');
  Product6 : Subsystem
      mask Display: disp('NFP\nmul');
  Product6_outbuff : hdlmdlgenlib/Buffer
      settings: SourceProductName=Simulink  SourceProductBaseCode=SL
  Product7 : Subsystem
      mask Display: disp('NFP\nmul');
  Product8 : Subsystem
      mask Display: disp('NFP\nmul');
  Product9 : Subsystem
      mask Display: disp('NFP\nmul');
  Product9_outbuff : hdlmdlgenlib/Buffer
      settings: SourceProductName=Simulink  SourceProductBaseCode=SL
  Sum : Subsystem
      mask Display: disp('NFP\nadd');
  Sum1 : Subsystem
      mask Display: disp('NFP\nadd');
  Sum10 : Subsystem
      mask Display: disp('NFP\nadd');
  Sum11 : Subsystem
      mask Display: disp('NFP\nadd');
  Sum11_outbuff : hdlmdlgenlib/Buffer
      settings: SourceProductName=Simulink  SourceProductBaseCode=SL
  Sum2 : Subsystem
      mask Display: disp('NFP\nadd');
  Sum3 : Subsystem
      mask Display: disp('NFP\nadd');
  Sum3_outbuff : hdlmdlgenlib/Buffer
      settings: SourceProductName=Simulink  SourceProductBaseCode=SL
  Sum4 : Subsystem
      mask Display: disp('NFP\nadd');
  Sum4_outbuff : hdlmdlgenlib/Buffer
      settings: SourceProductName=Simulink  SourceProductBaseCode=SL
  Sum5 : Subsystem
      mask Display: disp('NFP\nadd');
  Sum6 : Subsystem
      mask Display: disp('NFP\nadd');
  Sum7 : Subsystem
      mask Display: disp('NFP\nadd');
  Sum7_outbuff : hdlmdlgenlib/Buffer
      settings: SourceProductName=Simulink  SourceProductBaseCode=SL
  Sum8 : Subsystem
      mask Display: disp('NFP\nadd');
  Sum8_outbuff : hdlmdlgenlib/Buffer
      settings: SourceProductName=Simulink  SourceProductBaseCode=SL
  Sum9 : Subsystem
      mask Display: disp('NFP\nadd');
  Sum_outbuff : hdlmdlgenlib/Buffer
      settings: SourceProductName=Simulink  SourceProductBaseCode=SL
  Unit Delay{,1..7} (8 alike) : UnitDelay  InitialCondition=single(0)  SampleTime=2.08333333333333e-05
  output : Outport  VectorParamsAs1DForOutWhenUnconnected=off
  wires:
  Product15_to_gain/1(Out1) -> output/1
  Sum9/1(Out1) -> Sum10/2(In2)
  Sum8/1(Out1) -> Sum8_outbuff/1
  Sum7/1(Out1) -> Sum7_outbuff/1
  Sum6/1(Out1) -> Sum7/1(In1)
  Sum5/1(Out1) -> Sum6/2(In2)
  Sum4/1(Out1) -> Sum4_outbuff/1
  Sum3/1(Out1) -> Sum3_outbuff/1
  Sum2/1(Out1) -> Sum3/1(In1)
  Sum11/1(Out1) -> Sum11_outbuff/1
  Sum10/1(Out1) -> Sum11/1(In1)
  Sum1/1(Out1) -> Sum2/2(In2)
  Sum/1(Out1) -> Sum_outbuff/1
  Product9/1(Out1) -> Product9_outbuff/1
  Product8/1(Out1) -> Sum6/1(In1)
  Product7/1(Out1) -> Sum5/1(In1)
  Product6/1(Out1) -> Product6_outbuff/1
  Product5/1(Out1) -> Sum5/2(In2)
  Product4/1(Out1) -> Product4_outbuff/1
  Product3/1(Out1) -> Sum2/1(In1)
  Product2/1(Out1) -> Sum1/1(In1)
  Product14/1(Out1) -> Product14_outbuff/1
  Product13/1(Out1) -> Sum10/1(In1)
  Product12/1(Out1) -> Sum9/1(In1)
  Product11/1(Out1) -> Product11_outbuff/1
  Product10/1(Out1) -> Sum9/2(In2)
  Product1/1(Out1) -> Product1_outbuff/1
  Product/1(Out1) -> Sum1/2(In2)
  Gain8_unaryminus/1(Out1) -> Gain8_unaryminus_outbuff/1
  Gain7_unaryminus/1(Out1) -> Gain7_unaryminus_outbuff/1
  Gain5_unaryminus/1(Out1) -> Gain5_unaryminus_outbuff/1
  Gain3_unaryminus/1(Out1) -> Gain3_unaryminus_outbuff/1
  Gain2_unaryminus/1(Out1) -> Gain2_unaryminus_outbuff/1
  Gain1_unaryminus/1(Out1) -> Gain1_unaryminus_outbuff/1
  Unit Delay7/1 -> Gain8_unaryminus/1(In1)
  Unit Delay6/1 -> Unit Delay7/1, Gain7_unaryminus/1(In1)
  Unit Delay5/1 -> Gain5_unaryminus/1(In1), Product10/2(In2)
  Unit Delay4/1 -> Unit Delay5/1, Gain3_unaryminus/1(In1), Product12/2(In2)
  Unit Delay3/1 -> Gain2_unaryminus/1(In1), Product5/2(In2)
  Unit Delay2/1 -> Unit Delay3/1, Gain1_unaryminus/1(In1), Product7/2(In2)
  Unit Delay1/1 -> Product/2(In2)
  Unit Delay/1 -> Unit Delay1/1, Product2/2(In2)
  Sum8_outbuff/1 -> Sum11/2(In2)
  Sum7_outbuff/1 -> Unit Delay4/1, Product13/2(In2)
  Sum4_outbuff/1 -> Sum7/2(In2)
  Sum3_outbuff/1 -> Unit Delay2/1, Product8/2(In2)
  Sum11_outbuff/1 -> Unit Delay6/1, Product15_to_gain/1(In1)
  Sum_outbuff/1 -> Sum3/2(In2)
  Product9_outbuff/1 -> Sum4/1(In1)
  Product6_outbuff/1 -> Sum4/2(In2)
  Product4_outbuff/1 -> Sum/1(In1)
  Product14_outbuff/1 -> Sum8/1(In1)
  Product11_outbuff/1 -> Sum8/2(In2)
  Product1_outbuff/1 -> Sum/2(In2)
  Gain8_unaryminus_outbuff/1 -> Product11/2(In2)
  Gain7_unaryminus_outbuff/1 -> Product14/2(In2)
  Gain5_unaryminus_outbuff/1 -> Product6/2(In2)
  Gain3_unaryminus_outbuff/1 -> Product9/2(In2)
  Gain2_unaryminus_outbuff/1 -> Product1/2(In2)
  Gain1_unaryminus_outbuff/1 -> Product4/2(In2)
  Constant9/1 -> Product4/1(In1)
  Constant8/1 -> Product10/1(In1)
  Constant7/1 -> Product12/1(In1)
  Constant6/1 -> Product13/1(In1)
  Constant5/1 -> Product5/1(In1)
  Constant4/1 -> Product7/1(In1)
  Constant3/1 -> Product8/1(In1)
  Constant2/1 -> Product/1(In1)
  Constant14/1 -> Product11/1(In1)
  Constant13/1 -> Product6/1(In1)
  Constant12/1 -> Product14/1(In1)
  Constant11/1 -> Product9/1(In1)
  Constant10/1 -> Product1/1(In1)
  Constant1/1 -> Product2/1(In1)
  Constant/1 -> Product3/1(In1)
  stimulus/1 -> Unit Delay/1, Product3/2(In2)

== system AN_Simulink_Model_v1_fil/Auditory Nerve Model/Subsystem ==
  C2filterout : Inport  OutDataTypeStr=single  PortDimensions=1  SampleTime=2.08333333333333e-05
  C1filterout : Inport  Port=2  OutDataTypeStr=single  PortDimensions=1  SampleTime=2.08333333333333e-05
  IHC C1 NL Logarithmic Function : Subsystem
  IHC C2 NL Logarithmic Function : Subsystem
  IHC LP Filter : Subsystem
  Sum1 : Subsystem
      mask Display: disp('NFP\nadd');
  ihcout : Outport  VectorParamsAs1DForOutWhenUnconnected=off
  wires:
  Sum1/1(Out1) -> IHC LP Filter/1(stimulus)
  IHC LP Filter/1(output) -> ihcout/1
  IHC C2 NL Logarithmic Function/1(output) -> Sum1/1(In1)
  IHC C1 NL Logarithmic Function/1(output) -> Sum1/2(In2)
  C1filterout/1 -> IHC C1 NL Logarithmic Function/1(stimulus)
  C2filterout/1 -> IHC C2 NL Logarithmic Function/1(stimulus)

== system AN_Simulink_Model_v1_fil/Auditory Nerve Model/Subsystem1 ==
  wbout : Inport  OutDataTypeStr=single  PortDimensions=1  SampleTime=2.08333333333333e-05
  Calculate tauc1 : Subsystem
  NL After OHC Function : Subsystem
  OHC LP Filter : Subsystem
  OHC NL Boltzman Function : Subsystem
  tauc1 : Outport  VectorParamsAs1DForOutWhenUnconnected=off
  wires:
  OHC NL Boltzman Function/1(output) -> OHC LP Filter/1(stimulus)
  OHC LP Filter/1(output) -> NL After OHC Function/1(stimulus)
  NL After OHC Function/1(output) -> Calculate tauc1/1(In1)
  Calculate tauc1/1(Out1) -> tauc1/1
  wbout/1 -> OHC NL Boltzman Function/1(stimulus)

== system AN_Simulink_Model_v1_fil/Compare/Assert_ihcout ==
  cosim : Inport
  dut : Inport  Port=2
  AssertEq : Assertion  StopWhenAssertionFail=off
  Compare To Zero : simulink/Logic and Bit Operations/Compare To Zero  relop===  OutDataTypeStr=boolean
  RelErrCheck : Subsystem
  compare: ihcout : Scope  NumInputPorts=3
  wires:
  dut/1 -> compare: ihcout/2, RelErrCheck/2(In2)  "dut ref"
  cosim/1 -> compare: ihcout/1, RelErrCheck/1(In1)  "cosim"
  RelErrCheck/1(Out1) -> AssertEq/1, Compare To Zero/1
  Compare To Zero/1 -> compare: ihcout/3  "err"

== system AN_Simulink_Model_v1_fil/Compare/CleanupScopes ==

== system AN_Simulink_Model_v1_fil/Compare/Enable ==
